simulink library "CPTLibrary"  (R2018a)
settings: Solver=VariableStepAuto  StartTime=0.0  StopTime=10.0  RelTol=1e-3
undefined symbols (not defined in the file or in its folder): DiscIntNeverNeededParam
libraries: $bdroot x28
settings Model: Creator=daniemot  LastModifiedBy=daniemot

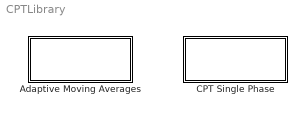
== system CPTLibrary ==
  Adaptive Moving Averages : Subsystem
  CPT Single Phase : Subsystem

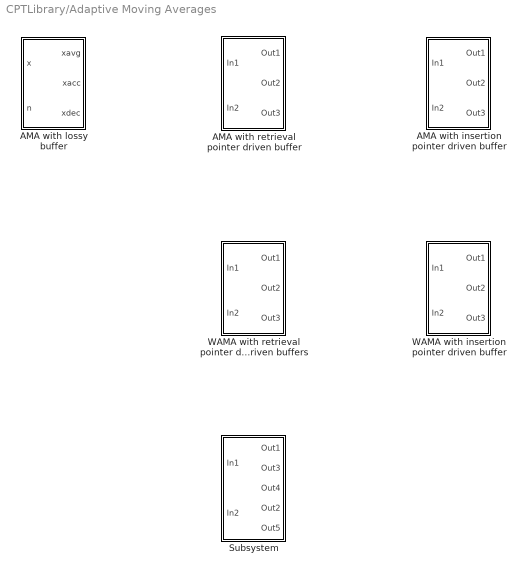
== system CPTLibrary/Adaptive Moving Averages ==
  AMA with insertion pointer driven buffer : Subsystem  TreatAsAtomicUnit=on  SystemSampleTime=Ts  mask(AMA with insertion pointer driven){NbSize=100, Ts=0.001}
      mask prompts: NbSize "Max number of samples for averaging"; Ts "Sampling time [s]"
      mask help:
      | Adaptive moving average with insertion pointer driven circular buffer
      |
      | Interface
      | Input	x (scalar): signal for averaging
      | 	n (scalar): number of previous samples of the input to be averaged with the current input
      | Output	xavg (scalar): average of the current input and the last n-samples of the input.
      | 	xacc (scalar): internal value sent for accumulation
      | 	xdec (scalar): internal value sent for decumulation
      | Parameters	nmax (scalar): maximum length of the length of the circular buffer
      | 	Ts (scalar): sampling time in [s]
      | Internal circular buffer:
      | 	Insertion pointer: i, always marches forward, x(now) replaces the slot pointed by i
      | 	Retrieval pointer: r, lags i by n samples, zeros the slot once retrieved, allowed to jump backwards, collects all values for decumulation and zeros slots when jumping forward.
      |
      | Prog/rev. semi-history:
      | 	Mota, 2020-11-24: first release
  AMA with lossy buffer : Subsystem  TreatAsAtomicUnit=on  SystemSampleTime=Ts  mask(AMA with a skipping circular buffer.){NbSize=100, Ts=0.001}
      mask prompts: NbSize "Max number of samples for averaging"; Ts "Sampling time [s]"
      mask help:
      | Adaptive moving average built with Matlab's discrete variable time delay
      |
      | Interface
      | Input	x (scalar): signal for averaging
      | 	n (scalar): number of previous samples of the input to be averaged with the current input
      | Output	xavg (scalar): average of the current input and the last n-samples of the input.
      | 	xacc (scalar): internal value sent for accumulation
      | 	xdec (scalar): internal value sent for decumulation
      | Parameters	nmax (scalar): maximum length of the length of the circular buffer
      | 	Ts (scalar): sampling time in [s]
      | Internal circular buffer:
      | 	Matlab's variable discrete time delay
      | 	Skips/double decumulations when n changes
      |
      | Prog/rev. semi-history:
      | 	Mota, 2020-11-24: first release
  AMA with retrieval pointer driven buffer : Subsystem  TreatAsAtomicUnit=on  SystemSampleTime=Ts  mask(AMA with retrieval pointer driven buffer){NbSize=100, Ts=0.001}
      mask prompts: NbSize "Max number of samples for averaging"; Ts "Sampling time [s]"
      mask help:
      | Adaptive moving average with retrieval poitner driven circular buffer
      |
      | Interface
      | Input	x (scalar): signal for averaging
      | 	n (scalar): number of previous samples of the input to be averaged with the current input
      | Output	xavg (scalar): average of the current input and the last n-samples of the input.
      | 	xacc (scalar): internal value sent for accumulation
      | 	xdec (scalar): internal value sent for decumulation
      | Parameters	nmax (scalar): maximum length of the length of the circular buffer
      | 	Ts (scalar): sampling time in [s]
      | Internal circular buffer:
      | 	Retrieval pointer: r, always marches forward, zero the slot after retrieval.
      | 	Insertion pointer: i, marches n slots ahead of r, allowed to jump, sums x(now) to the whichever value present at the insertion slot
      |
      | Prog/rev. semi-history:
      | 	Mota, 2020-11-24: first release
  Subsystem : Subsystem  TreatAsAtomicUnit=on  SystemSampleTime=Ts  mask(HAMA with retrieval pointer driven buffer){NbSize=100, Ts=0.001}
      mask prompts: NbSize "Max number of samples for averaging"; Ts "Sampling time [s]"
      mask help:
      | Hybrid adaptive moving average with three retrieval pointer driven circular buffers.
      |
      | Interface
      | Input	x (scalar): signal for averaging
      | 	n (scalar): number of previous samples of the input to be averaged with the current input
      | Output	xavg (scalar): average of the current input and the last hybrid number of 'n'-samples of the input.
      | 	xavground (scalar): average of the current input and the last round(n)-samples of the input.
      | 	xavgceil (scalar): average of the current input and the last ceil(n)-samples of the input.
      | 	xavgfloor (scalar): average of the current input and the last floor(n)-samples of the input.
      | 	xavgweighed (scalar): average of the current input and the last weighted(n)-samples of the input.
      | Parameters	nmax (scalar): maximum length of the length of the circular buffer
      | 	Ts (scalar): sampling time in [s]
      |
      | Prog/rev. semi-history:
      | 	Mota, 2020-12-08: first release
  WAMA with insertion pointer driven buffer : Subsystem  TreatAsAtomicUnit=on  SystemSampleTime=Ts  mask(WAMA with insertion pointer driven buffer){NbSize=0, Ts=0}
      mask prompts: NbSize "Max number of samples for averaging"; Ts "Sampling time [s]"
      mask help:
      | Adaptive moving average with two insertion pointer driven circular buffers.
      |
      | Interface
      | Input	x (scalar): signal for averaging
      | 	n (scalar): number of previous samples of the input to be averaged with the current input
      | Output	xavg (scalar): weigthed average of the current input and the last 'n'-samples of the input.
      | 	xavgceil (scalar): average of the current input and the last ceil(n)-samples of the input.
      | 	xavgfloor (scalar): average of the current input and the last floor(n)-samples of the input.
      | Parameters	nmax (scalar): maximum length of the length of the circular buffer
      | 	Ts (scalar): sampling time in [s]
      |
      | Prog/rev. semi-history:
      | 	Mota, 2020-11-24: first release
  WAMA with retrieval pointer driven buffers : Subsystem  TreatAsAtomicUnit=on  SystemSampleTime=Ts  mask(WAMA with retrieval pointer driven buffer){NbSize=100, Ts=0.001}
      mask prompts: NbSize "Max number of samples for averaging"; Ts "Sampling time [s]"
      mask help:
      | Adaptive moving average with two retrieval pointer driven circular buffers.
      |
      | Interface
      | Input	x (scalar): signal for averaging
      | 	n (scalar): number of previous samples of the input to be averaged with the current input
      | Output	xavg (scalar): weigthed average of the current input and the last 'n'-samples of the input.
      | 	xavgceil (scalar): average of the current input and the last ceil(n)-samples of the input.
      | 	xavgfloor (scalar): average of the current input and the last floor(n)-samples of the input.
      | Parameters	nmax (scalar): maximum length of the length of the circular buffer
      | 	Ts (scalar): sampling time in [s]
      |
      | Prog/rev. semi-history:
      | 	Mota, 2020-11-24: first release

== system CPTLibrary/CPT Single Phase ==
  Single phase CPT Lossy AMA : Subsystem  TreatAsAtomicUnit=on  SystemSampleTime=Ts  mask(Single phase CPT transducer with Skipping AMAs){NbSize=100, Ts=0.001}
      mask prompts: NbSize "Maximum number of samples per period"; Ts "Sampling time [s]"
      mask help:
      | Input	Voltage: v, scalar
      | 	Current: i, scalar
      | 	Frequecy: f, scalar in [Hz]
      | Output	Active power: p
      | 	Active current: ia
      | 	Reactive power: q
      | 	Reactive energy: w
      | 	Reactive current: ir
      | 	Void current: iv
      | 	Integral of the voltage: vint
      | 	Bias of the int. of the volt.: vintbias
      | 	Voltage times current: vi
      | 	Unbiased int. voltage times current: vinthati
      | Parameters	nmax (scalar): maximum length of the length of the circular buffers
      | 	Ts (scalar): sampling time in [s]
      |
      | Prog/rev. semi-history:
      | 	Mota, 2020-11-24: first release
      | 	Mota, 2020-12-08: added voltages and currents to interface
  Single phase CPT Retrieval AMA : Subsystem  TreatAsAtomicUnit=on  SystemSampleTime=Ts  mask(Single Phase CPT Retrieval AMAs){NbSize=100, Ts=0.001}
      mask prompts: NbSize "Maximum number of samples per period"; Ts "Sampling time [s]"
      mask help:
      | Input	Voltage: v, scalar
      | 	Current: i, scalar
      | 	Frequecy: f, scalar in [Hz]
      | Output	Active power: p
      | 	Active current: ia
      | 	Reactive power: q
      | 	Reactive energy: w
      | 	Reactive current: ir
      | 	Void current: iv
      | 	Integral of the voltage: vint
      | 	Bias of the int. of the volt.: vintbias
      | 	Voltage times current: vi
      | 	Unbiased int. voltage times current: vinthati
      | Parameters	nmax (scalar): maximum length of the length of the circular buffers
      | 	Ts (scalar): sampling time in [s]
      |
      | Prog/rev. semi-history:
      | 	Mota, 2020-11-24: first release
      | 	Mota, 2020-12-08: added voltages and currents to interface
  Single phase CPT Retrieval HAMA : Subsystem  TreatAsAtomicUnit=on  SystemSampleTime=Ts  mask{NbSize=100, Ts=0.001}
      mask prompts: NbSize "Maximum number of samples per period"; Ts "Sampling time [s]"
      mask help:
      | Input	Voltage: v, scalar
      | 	Current: i, scalar
      | 	Frequecy: f, scalar in [Hz]
      | Output	Active power: p
      | 	Active current: ia
      | 	Reactive power: q
      | 	Reactive energy: w
      | 	Reactive current: ir
      | 	Void current: iv
      | 	Integral of the voltage: vint
      | 	Bias of the int. of the volt.: vintbias
      | 	Voltage times current: vi
      | 	Unbiased int. voltage times current: vinthati
      | Parameters	nmax (scalar): maximum length of the length of the circular buffers
      | 	Ts (scalar): sampling time in [s]
      |
      | Prog/rev. semi-history:
      | 	Mota, 2020-12-08: first release
  Single phase CPT Retrieval WAMA : Subsystem  TreatAsAtomicUnit=on  SystemSampleTime=Ts  mask(Single phase CPT with Retrieval WAMAs){NbSize=100, Ts=0.001}
      mask prompts: NbSize "Maximum number of samples per period"; Ts "Sampling time [s]"
      mask help:
      | Input	Voltage: v, scalar
      | 	Current: i, scalar
      | 	Frequecy: f, scalar in [Hz]
      | Output	Active power: p
      | 	Active current: ia
      | 	Reactive power: q
      | 	Reactive energy: w
      | 	Reactive current: ir
      | 	Void current: iv
      | 	Integral of the voltage: vint
      | 	Bias of the int. of the volt.: vintbias
      | 	Voltage times current: vi
      | 	Unbiased int. voltage times current: vinthati
      | Parameters	nmax (scalar): maximum length of the length of the circular buffers
      | 	Ts (scalar): sampling time in [s]
      |
      | Prog/rev. semi-history:
      | 	Mota, 2020-11-24: first release
      | 	Mota, 2020-12-08: added voltages and currents to interface

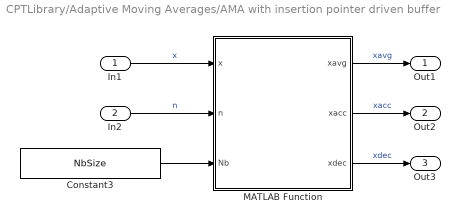
== system CPTLibrary/Adaptive Moving Averages/AMA with insertion pointer driven buffer ==
  In1 : Inport
  In2 : Inport  Port=2
  Constant3 : Constant  Value=NbSize
  MATLAB Function : MATLAB Function  TreatAsAtomicUnit=on
  Out1 : Outport
  Out2 : Outport  Port=2
  Out3 : Outport  Port=3
  wires:
  In2/1 -> MATLAB Function/2(n)  "n"
  MATLAB Function/1(xavg) -> Out1/1  "xavg"
  Constant3/1 -> MATLAB Function/3(Nb)
  MATLAB Function/2(xacc) -> Out2/1  "xacc"
  MATLAB Function/3(xdec) -> Out3/1  "xdec"
  In1/1 -> MATLAB Function/1(x)  "x"

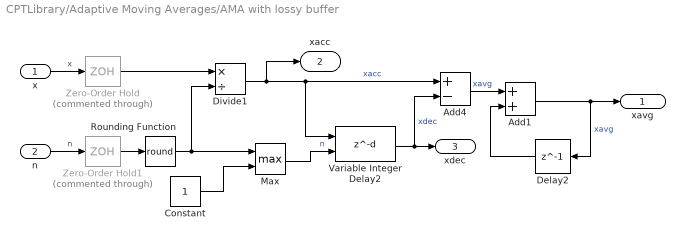
== system CPTLibrary/Adaptive Moving Averages/AMA with lossy buffer ==
  x : Inport
  n : Inport  Port=2
  Add1 : Sum
  Add4 : Sum  Inputs=+-
  Constant : Constant
  Delay2 : Delay  DelayLength=1  InitialCondition=0  UseCircularBuffer=on  SampleTime=Ts
  Divide1 : Product  Inputs=*/
  Max : MinMax  Function=max  Inputs=2
  Rounding Function : Rounding  Operator=round
  Variable Integer Delay2 : Delay  DelayLengthSource=Input port  DelayLengthUpperLimit=NbSize  UseCircularBuffer=on  SampleTime=Ts
      settings: InputPortMap=u0,p1
  Zero-Order Hold : ZeroOrderHold  Commented=through  SampleTime=Ts
  Zero-Order Hold1 : ZeroOrderHold  Commented=through  SampleTime=Ts
  xavg : Outport
  xacc : Outport  Port=2
  xdec : Outport  Port=3
  wires:
  n/1 -> Zero-Order Hold1/1  "n"
  x/1 -> Zero-Order Hold/1  "x"
  Divide1/1 -> Add4/1, Variable Integer Delay2/1, xacc/1  "xacc"
  Variable Integer Delay2/1 -> Add4/2, xdec/1  "xdec"
  Constant/1 -> Max/2
  Max/1 -> Variable Integer Delay2/2  "n"
  Add4/1 -> Add1/1  "xavg"
  Add1/1 -> Delay2/1, xavg/1  "xavg"
  Delay2/1 -> Add1/2
  Zero-Order Hold/1 -> Divide1/1
  Zero-Order Hold1/1 -> Rounding Function/1
  Rounding Function/1 -> Divide1/2, Max/1

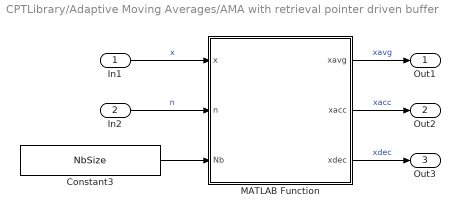
== system CPTLibrary/Adaptive Moving Averages/AMA with retrieval pointer driven buffer ==
  In1 : Inport
  In2 : Inport  Port=2
  Constant3 : Constant  Value=NbSize
  MATLAB Function : MATLAB Function  TreatAsAtomicUnit=on
  Out1 : Outport
  Out2 : Outport  Port=2
  Out3 : Outport  Port=3
  wires:
  MATLAB Function/3(xdec) -> Out3/1  "xdec"
  MATLAB Function/1(xavg) -> Out1/1  "xavg"
  Constant3/1 -> MATLAB Function/3(Nb)
  In1/1 -> MATLAB Function/1(x)  "x"
  In2/1 -> MATLAB Function/2(n)  "n"
  MATLAB Function/2(xacc) -> Out2/1  "xacc"

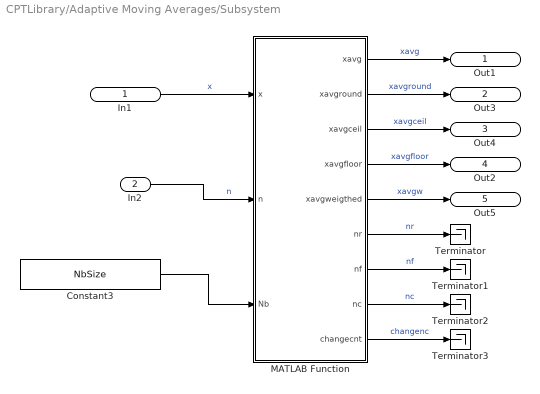
== system CPTLibrary/Adaptive Moving Averages/Subsystem ==
  In1 : Inport
  In2 : Inport  Port=2
  Constant3 : Constant  Value=NbSize
  MATLAB Function : MATLAB Function  TreatAsAtomicUnit=on
  Terminator{,1..3} (4 alike) : Terminator
  Out1 : Outport
  Out3 : Outport  Port=2
  Out4 : Outport  Port=3
  Out2 : Outport  Port=4
  Out5 : Outport  Port=5
  wires:
  MATLAB Function/1(xavg) -> Out1/1  "xavg"
  MATLAB Function/2(xavground) -> Out3/1  "xavground"
  MATLAB Function/3(xavgceil) -> Out4/1  "xavgceil"
  MATLAB Function/4(xavgfloor) -> Out2/1  "xavgfloor"
  MATLAB Function/6(nr) -> Terminator/1  "nr"
  MATLAB Function/7(nf) -> Terminator1/1  "nf"
  MATLAB Function/8(nc) -> Terminator2/1  "nc"
  MATLAB Function/9(changecnt) -> Terminator3/1  "changenc"
  In1/1 -> MATLAB Function/1(x)  "x"
  Constant3/1 -> MATLAB Function/3(Nb)
  In2/1 -> MATLAB Function/2(n)  "n"
  MATLAB Function/5(xavgweigthed) -> Out5/1  "xavgw"

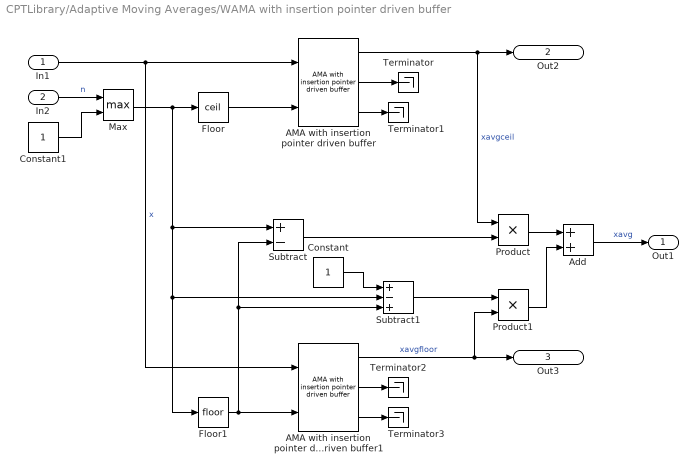
== system CPTLibrary/Adaptive Moving Averages/WAMA with insertion pointer driven buffer ==
  In1 : Inport
  In2 : Inport  Port=2
  AMA with insertion pointer driven buffer : $bdroot/Adaptive Moving Averages/AMA with insertion pointer driven buffer  NbSize=NbSize  Ts=Ts
  AMA with insertion pointer driven buffer1 : $bdroot/Adaptive Moving Averages/AMA with insertion pointer driven buffer  NbSize=NbSize  Ts=Ts
  Add : Sum
  Constant : Constant
  Constant1 : Constant
  Floor : Rounding  Operator=ceil
  Floor1 : Rounding
  Max : MinMax  Function=max  Inputs=2
  Product : Product
  Product1 : Product
  Subtract : Sum  Inputs=+-
  Subtract1 : Sum  Inputs=+-+
  Terminator{,1..3} (4 alike) : Terminator
  Out1 : Outport
  Out2 : Outport  Port=2
  Out3 : Outport  Port=3
  wires:
  AMA with insertion pointer driven buffer/1 -> Out2/1, Product/1  "xavgceil"
  AMA with insertion pointer driven buffer/2 -> Terminator/1
  Floor1/1 -> AMA with insertion pointer driven buffer1/2, Subtract1/3, Subtract/2
  Product1/1 -> Add/2
  Subtract/1 -> Product/2
  Product/1 -> Add/1
  Add/1 -> Out1/1  "xavg"
  Subtract1/1 -> Product1/1
  AMA with insertion pointer driven buffer1/2 -> Terminator2/1
  AMA with insertion pointer driven buffer1/3 -> Terminator3/1
  Floor/1 -> AMA with insertion pointer driven buffer/2
  AMA with insertion pointer driven buffer1/1 -> Product1/2, Out3/1  "xavgfloor"
  AMA with insertion pointer driven buffer/3 -> Terminator1/1
  Constant1/1 -> Max/2
  Max/1 -> Floor1/1, Subtract1/2, Subtract/1, Floor/1
  In2/1 -> Max/1  "n"
  Constant/1 -> Subtract1/1
  In1/1 -> AMA with insertion pointer driven buffer1/1, AMA with insertion pointer driven buffer/1  "x"

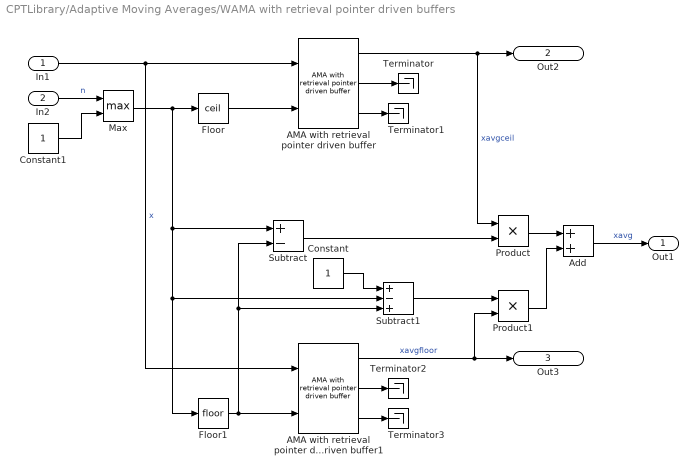
== system CPTLibrary/Adaptive Moving Averages/WAMA with retrieval pointer driven buffers ==
  In1 : Inport
  In2 : Inport  Port=2
  AMA with retrieval pointer driven buffer : $bdroot/Adaptive Moving Averages/AMA with retrieval pointer driven buffer  NbSize=NbSize  Ts=Ts
  AMA with retrieval pointer driven buffer1 : $bdroot/Adaptive Moving Averages/AMA with retrieval pointer driven buffer  NbSize=NbSize  Ts=Ts
  Add : Sum
  Constant : Constant
  Constant1 : Constant
  Floor : Rounding  Operator=ceil
  Floor1 : Rounding
  Max : MinMax  Function=max  Inputs=2
  Product : Product
  Product1 : Product
  Subtract : Sum  Inputs=+-
  Subtract1 : Sum  Inputs=+-+
  Terminator{,1..3} (4 alike) : Terminator
  Out1 : Outport
  Out2 : Outport  Port=2
  Out3 : Outport  Port=3
  wires:
  AMA with retrieval pointer driven buffer/3 -> Terminator1/1
  In1/1 -> AMA with retrieval pointer driven buffer1/1, AMA with retrieval pointer driven buffer/1  "x"
  Floor1/1 -> AMA with retrieval pointer driven buffer1/2, Subtract1/3, Subtract/2
  AMA with retrieval pointer driven buffer/2 -> Terminator/1
  Product1/1 -> Add/2
  Subtract1/1 -> Product1/1
  Add/1 -> Out1/1  "xavg"
  Product/1 -> Add/1
  Subtract/1 -> Product/2
  AMA with retrieval pointer driven buffer/1 -> Out2/1, Product/1  "xavgceil"
  Floor/1 -> AMA with retrieval pointer driven buffer/2
  In2/1 -> Max/1  "n"
  AMA with retrieval pointer driven buffer1/2 -> Terminator2/1
  Constant/1 -> Subtract1/1
  AMA with retrieval pointer driven buffer1/1 -> Product1/2, Out3/1  "xavgfloor"
  AMA with retrieval pointer driven buffer1/3 -> Terminator3/1
  Constant1/1 -> Max/2
  Max/1 -> Floor1/1, Subtract1/2, Subtract/1, Floor/1

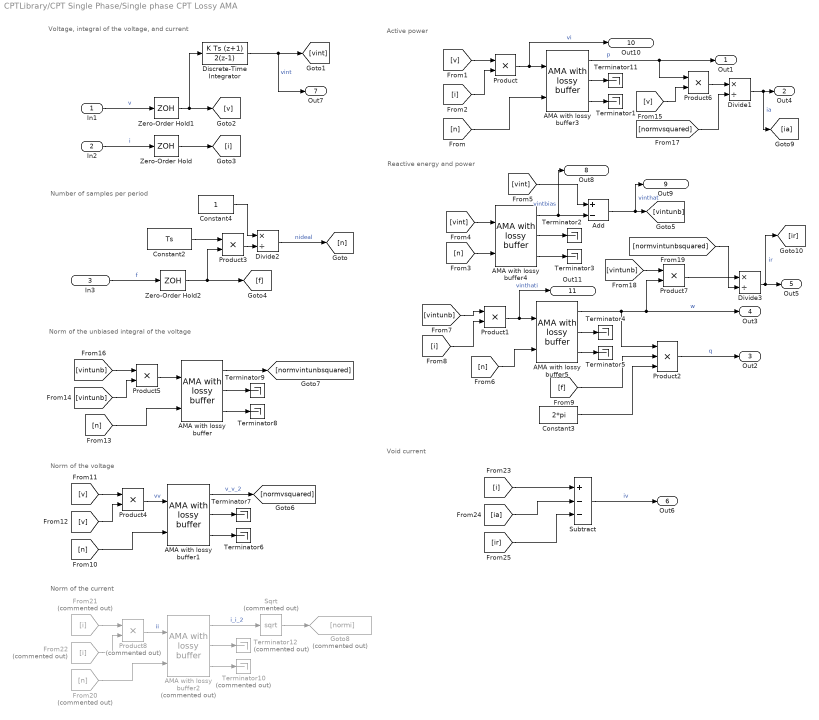
== system CPTLibrary/CPT Single Phase/Single phase CPT Lossy AMA ==
  note: Voltage, integral of the voltage, and current
  note: Number of samples per period
  note: Norm of the unbiased integral of the voltage
  note: Norm of the voltage
  note: Active power
  note: Reactive energy and power
  note: Norm of the current
  note: Void current
  In1 : Inport
  In2 : Inport  Port=2
  In3 : Inport  Port=3
  AMA with lossy buffer{,1,3..5} (5 alike) : $bdroot/Adaptive Moving Averages/AMA with lossy buffer  NbSize=NbSize  Ts=Ts
  AMA with lossy buffer2 : $bdroot/Adaptive Moving Averages/AMA with lossy buffer  Commented=on  NbSize=NbSize  Ts=Ts
  Add : Sum  Inputs=+-
  Constant2 : Constant  Value=Ts
  Constant3 : Constant  Value=2*pi
  Constant4 : Constant
  Discrete-Time Integrator : DiscreteIntegrator  IntegratorMethod=Integration: Trapezoidal  SampleTime=Ts  ICPrevOutput=DiscIntNeverNeededParam  ICPrevScaledInput=DiscIntNeverNeededParam
  Divide1 : Product  Inputs=*/
  Divide2 : Product  Inputs=*/
  Divide3 : Product  Inputs=*/
  From20 : From  Commented=on  GotoTag=n
  From21 : From  Commented=on  GotoTag=i
  From22 : From  Commented=on  GotoTag=i
  Goto8 : Goto  Commented=on  GotoTag=normi
  Product{,1,3..7} (7 alike) : Product
  Product2 : Product  Inputs=3
  Product8 : Product  Commented=on
  Sqrt : Sqrt  Commented=on  SaturateOnIntegerOverflow=on
  Subtract : Sum  Inputs=+--
  Terminator{1..9,11} (10 alike) : Terminator
  Terminator10 : Terminator  Commented=on
  Terminator12 : Terminator  Commented=on
  Zero-Order Hold : ZeroOrderHold  SampleTime=Ts
  Zero-Order Hold1 : ZeroOrderHold  SampleTime=Ts
  Zero-Order Hold2 : ZeroOrderHold  SampleTime=Ts
  Out1 : Outport
  Out4 : Outport  Port=2
  Out2 : Outport  Port=3
  Out3 : Outport  Port=4
  Out5 : Outport  Port=5
  Out6 : Outport  Port=6
  Out7 : Outport  Port=7
  Out8 : Outport  Port=8
  Out9 : Outport  Port=9
  Out10 : Outport  Port=10
  Out11 : Outport  Port=11
  wires:
  [n] -> AMA with lossy buffer3/2
  AMA with lossy buffer3/2 -> Terminator11/1
  AMA with lossy buffer3/3 -> Terminator1/1
  Product1/1 -> Out11/1, AMA with lossy buffer5/1  "vinthati"
  AMA with lossy buffer4/1 -> Out8/1, Add/2  "vintbias"
  AMA with lossy buffer4/2 -> Terminator2/1
  [n] -> AMA with lossy buffer4/2
  AMA with lossy buffer5/3 -> Terminator5/1
  AMA with lossy buffer4/3 -> Terminator3/1
  [n] -> AMA with lossy buffer5/2
  AMA with lossy buffer5/1 -> Product7/2, Out3/1, Product2/1  "w"
  [i] -> Product/2
  In1/1 -> Zero-Order Hold1/1  "v"
  In2/1 -> Zero-Order Hold/1  "i"
  [vint] -> Add/1
  Constant4/1 -> Divide2/1
  Divide2/1 -> [n]  "nideal"
  Product3/1 -> Divide2/2
  [v] -> Product/1
  Constant2/1 -> Product3/1
  AMA with lossy buffer5/2 -> Terminator4/1
  [f] -> Product2/2
  Constant3/1 -> Product2/3
  [i] -> Product1/2
  [vint] -> AMA with lossy buffer4/1
  Zero-Order Hold1/1 -> [v], Discrete-Time Integrator/1
  AMA with lossy buffer3/1 -> Product6/1, Out1/1  "p"
  [vintunb] -> Product1/1
  In3/1 -> Zero-Order Hold2/1  "f"
  Product/1 -> Out10/1, AMA with lossy buffer3/1  "vi"
  Zero-Order Hold2/1 -> Product3/2, [f]
  Zero-Order Hold/1 -> [i]
  Product2/1 -> Out2/1  "q"
  Discrete-Time Integrator/1 -> Out7/1, [vint]  "vint"
  Add/1 -> Out9/1, [vintunb]  "vinthat"
  AMA with lossy buffer1/3 -> Terminator6/1
  AMA with lossy buffer1/2 -> Terminator7/1
  AMA with lossy buffer1/1 -> [normvsquared]  "v_v_2"
  [v] -> Product4/1
  [n] -> AMA with lossy buffer1/2
  Product4/1 -> AMA with lossy buffer1/1  "vv"
  [v] -> Product4/2
  [n] -> AMA with lossy buffer/2
  AMA with lossy buffer/2 -> Terminator9/1
  AMA with lossy buffer/1 -> [normvintunbsquared]
  [vintunb] -> Product5/1
  Product5/1 -> AMA with lossy buffer/1
  AMA with lossy buffer/3 -> Terminator8/1
  [vintunb] -> Product5/2
  [v] -> Product6/2
  Product6/1 -> Divide1/1
  [normvsquared] -> Divide1/2
  Divide1/1 -> [ia], Out4/1  "ia"
  [vintunb] -> Product7/1
  Product7/1 -> Divide3/1
  [normvintunbsquared] -> Divide3/2
  Divide3/1 -> [ir], Out5/1  "ir"
  From20/1 -> AMA with lossy buffer2/2
  AMA with lossy buffer2/2 -> Terminator12/1
  AMA with lossy buffer2/1 -> Sqrt/1  "i_i_2"
  From21/1 -> Product8/1
  Product8/1 -> AMA with lossy buffer2/1  "ii"
  AMA with lossy buffer2/3 -> Terminator10/1
  From22/1 -> Product8/2
  Sqrt/1 -> Goto8/1
  [i] -> Subtract/1
  [ia] -> Subtract/2
  [ir] -> Subtract/3
  Subtract/1 -> Out6/1  "iv"

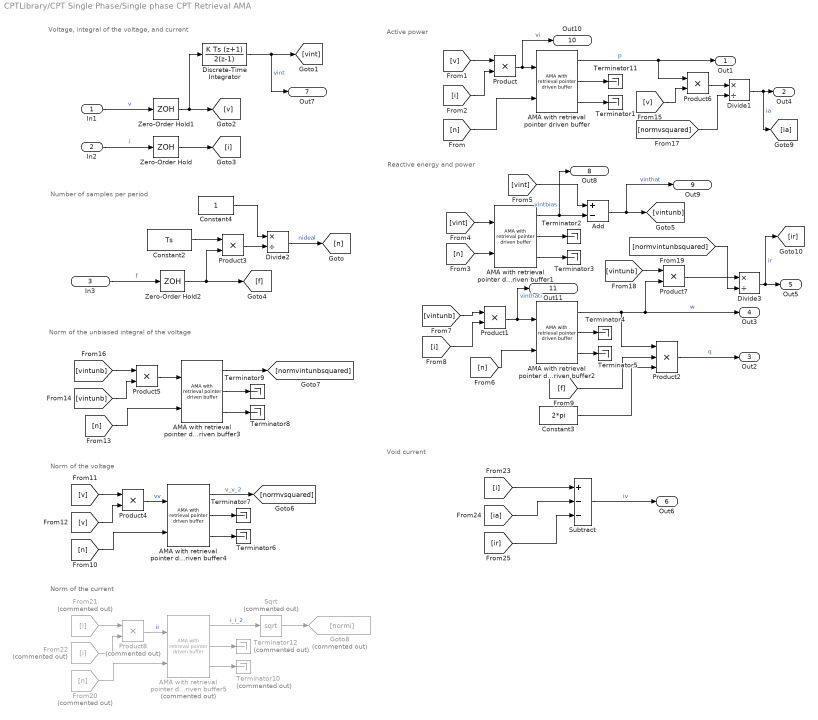
== system CPTLibrary/CPT Single Phase/Single phase CPT Retrieval AMA ==
  note: Norm of the voltage
  note: Void current
  note: Active power
  note: Norm of the current
  note: Number of samples per period
  note: Norm of the unbiased integral of the voltage
  note: Reactive energy and power
  note: Voltage, integral of the voltage, and current
  In1 : Inport
  In2 : Inport  Port=2
  In3 : Inport  Port=3
  AMA with retrieval pointer driven buffer{,1..4} (5 alike) : $bdroot/Adaptive Moving Averages/AMA with retrieval pointer driven buffer  NbSize=NbSize  Ts=Ts
  AMA with retrieval pointer driven buffer5 : $bdroot/Adaptive Moving Averages/AMA with retrieval pointer driven buffer  Commented=on  NbSize=NbSize  Ts=Ts
  Add : Sum  Inputs=+-
  Constant2 : Constant  Value=Ts
  Constant3 : Constant  Value=2*pi
  Constant4 : Constant
  Discrete-Time Integrator : DiscreteIntegrator  IntegratorMethod=Integration: Trapezoidal  SampleTime=Ts  ICPrevOutput=DiscIntNeverNeededParam  ICPrevScaledInput=DiscIntNeverNeededParam
  Divide1 : Product  Inputs=*/
  Divide2 : Product  Inputs=*/
  Divide3 : Product  Inputs=*/
  From20 : From  Commented=on  GotoTag=n
  From21 : From  Commented=on  GotoTag=i
  From22 : From  Commented=on  GotoTag=i
  Goto8 : Goto  Commented=on  GotoTag=normi
  Product{,1,3..7} (7 alike) : Product
  Product2 : Product  Inputs=3
  Product8 : Product  Commented=on
  Sqrt : Sqrt  Commented=on  SaturateOnIntegerOverflow=on
  Subtract : Sum  Inputs=+--
  Terminator{1..9,11} (10 alike) : Terminator
  Terminator10 : Terminator  Commented=on
  Terminator12 : Terminator  Commented=on
  Zero-Order Hold : ZeroOrderHold  SampleTime=Ts
  Zero-Order Hold1 : ZeroOrderHold  SampleTime=Ts
  Zero-Order Hold2 : ZeroOrderHold  SampleTime=Ts
  Out1 : Outport
  Out4 : Outport  Port=2
  Out2 : Outport  Port=3
  Out3 : Outport  Port=4
  Out5 : Outport  Port=5
  Out6 : Outport  Port=6
  Out7 : Outport  Port=7
  Out8 : Outport  Port=8
  Out9 : Outport  Port=9
  Out10 : Outport  Port=10
  Out11 : Outport  Port=11
  wires:
  AMA with retrieval pointer driven buffer2/1 -> Product7/2, Out3/1, Product2/1  "w"
  [n] -> AMA with retrieval pointer driven buffer2/2
  [n] -> AMA with retrieval pointer driven buffer1/2
  [i] -> Subtract/1
  AMA with retrieval pointer driven buffer2/3 -> Terminator5/1
  AMA with retrieval pointer driven buffer/2 -> Terminator11/1
  AMA with retrieval pointer driven buffer/1 -> Product6/1, Out1/1  "p"
  Product4/1 -> AMA with retrieval pointer driven buffer4/1  "vv"
  [ia] -> Subtract/2
  [vintunb] -> Product5/1
  Divide3/1 -> [ir], Out5/1  "ir"
  From22/1 -> Product8/2
  Product8/1 -> AMA with retrieval pointer driven buffer5/1  "ii"
  AMA with retrieval pointer driven buffer5/3 -> Terminator10/1
  From21/1 -> Product8/1
  Divide1/1 -> [ia], Out4/1  "ia"
  [normvintunbsquared] -> Divide3/2
  Product7/1 -> Divide3/1
  [n] -> AMA with retrieval pointer driven buffer4/2
  Sqrt/1 -> Goto8/1
  [vintunb] -> Product7/1
  Product1/1 -> Out11/1, AMA with retrieval pointer driven buffer2/1  "vinthati"
  [v] -> Product6/2
  AMA with retrieval pointer driven buffer3/1 -> [normvintunbsquared]
  [normvsquared] -> Divide1/2
  AMA with retrieval pointer driven buffer3/2 -> Terminator9/1
  AMA with retrieval pointer driven buffer2/2 -> Terminator4/1
  AMA with retrieval pointer driven buffer4/1 -> [normvsquared]  "v_v_2"
  [n] -> AMA with retrieval pointer driven buffer3/2
  AMA with retrieval pointer driven buffer4/2 -> Terminator7/1
  Discrete-Time Integrator/1 -> Out7/1, [vint]  "vint"
  Zero-Order Hold/1 -> [i]
  In3/1 -> Zero-Order Hold2/1  "f"
  AMA with retrieval pointer driven buffer/3 -> Terminator1/1
  Zero-Order Hold1/1 -> [v], Discrete-Time Integrator/1
  [vintunb] -> Product1/1
  [i] -> Product1/2
  Constant3/1 -> Product2/3
  [f] -> Product2/2
  [vint] -> Add/1
  [ir] -> Subtract/3
  Constant2/1 -> Product3/1
  Product3/1 -> Divide2/2
  Divide2/1 -> [n]  "nideal"
  [v] -> Product/1
  Zero-Order Hold2/1 -> Product3/2, [f]
  [i] -> Product/2
  In2/1 -> Zero-Order Hold/1  "i"
  In1/1 -> Zero-Order Hold1/1  "v"
  AMA with retrieval pointer driven buffer3/3 -> Terminator8/1
  From20/1 -> AMA with retrieval pointer driven buffer5/2
  Product5/1 -> AMA with retrieval pointer driven buffer3/1
  [n] -> AMA with retrieval pointer driven buffer/2
  [v] -> Product4/1
  [vint] -> AMA with retrieval pointer driven buffer1/1
  AMA with retrieval pointer driven buffer1/2 -> Terminator2/1
  Subtract/1 -> Out6/1  "iv"
  AMA with retrieval pointer driven buffer4/3 -> Terminator6/1
  Product6/1 -> Divide1/1
  AMA with retrieval pointer driven buffer5/1 -> Sqrt/1  "i_i_2"
  Add/1 -> Out9/1, [vintunb]  "vinthat"
  Product/1 -> Out10/1, AMA with retrieval pointer driven buffer/1  "vi"
  AMA with retrieval pointer driven buffer1/3 -> Terminator3/1
  Constant4/1 -> Divide2/1
  [v] -> Product4/2
  [vintunb] -> Product5/2
  Product2/1 -> Out2/1  "q"
  AMA with retrieval pointer driven buffer5/2 -> Terminator12/1
  AMA with retrieval pointer driven buffer1/1 -> Out8/1, Add/2  "vintbias"

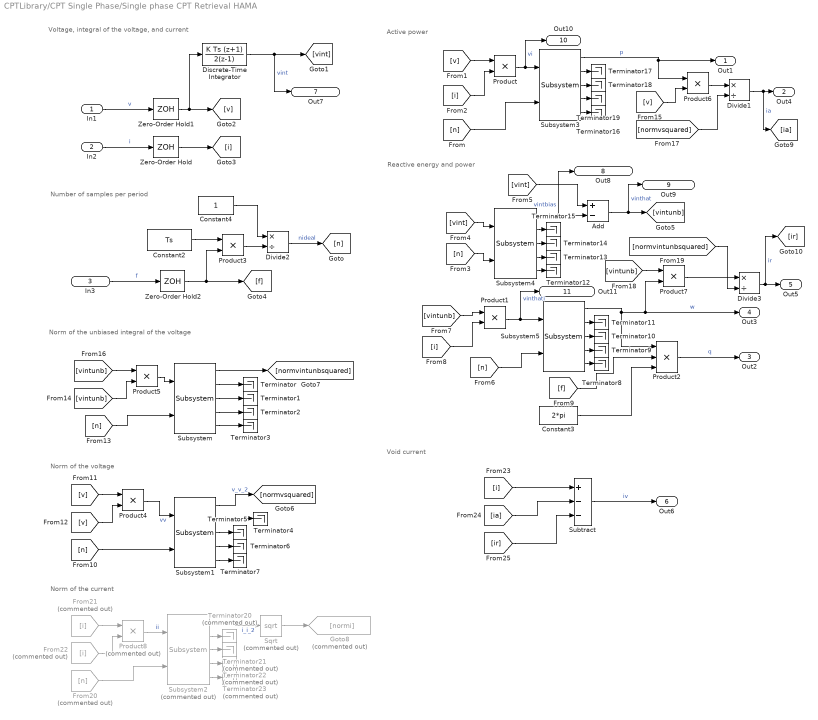
== system CPTLibrary/CPT Single Phase/Single phase CPT Retrieval HAMA ==
  note: Void current
  note: Number of samples per period
  note: Norm of the voltage
  note: Voltage, integral of the voltage, and current
  note: Reactive energy and power
  note: Active power
  note: Norm of the current
  note: Norm of the unbiased integral of the voltage
  In1 : Inport
  In2 : Inport  Port=2
  In3 : Inport  Port=3
  Add : Sum  Inputs=+-
  Constant2 : Constant  Value=Ts
  Constant3 : Constant  Value=2*pi
  Constant4 : Constant
  Discrete-Time Integrator : DiscreteIntegrator  IntegratorMethod=Integration: Trapezoidal  SampleTime=Ts  ICPrevOutput=DiscIntNeverNeededParam  ICPrevScaledInput=DiscIntNeverNeededParam
  Divide1 : Product  Inputs=*/
  Divide2 : Product  Inputs=*/
  Divide3 : Product  Inputs=*/
  From20 : From  Commented=on  GotoTag=n
  From21 : From  Commented=on  GotoTag=i
  From22 : From  Commented=on  GotoTag=i
  Goto8 : Goto  Commented=on  GotoTag=normi
  Product{,1,3..7} (7 alike) : Product
  Product2 : Product  Inputs=3
  Product8 : Product  Commented=on
  Sqrt : Sqrt  Commented=on  SaturateOnIntegerOverflow=on
  Subsystem{,1,3..5} (5 alike) : $bdroot/Adaptive Moving Averages/Subsystem  NbSize=NbSize  Ts=Ts
  Subsystem2 : $bdroot/Adaptive Moving Averages/Subsystem  Commented=on  NbSize=NbSize  Ts=Ts
  Subtract : Sum  Inputs=+--
  Terminator{,1..19} (20 alike) : Terminator
  Terminator{20..23} (4 alike) : Terminator  Commented=on
  Zero-Order Hold : ZeroOrderHold  SampleTime=Ts
  Zero-Order Hold1 : ZeroOrderHold  SampleTime=Ts
  Zero-Order Hold2 : ZeroOrderHold  SampleTime=Ts
  Out1 : Outport
  Out4 : Outport  Port=2
  Out2 : Outport  Port=3
  Out3 : Outport  Port=4
  Out5 : Outport  Port=5
  Out6 : Outport  Port=6
  Out7 : Outport  Port=7
  Out8 : Outport  Port=8
  Out9 : Outport  Port=9
  Out10 : Outport  Port=10
  Out11 : Outport  Port=11
  wires:
  Product6/1 -> Divide1/1
  [i] -> Product/2
  Product3/1 -> Divide2/2
  Product7/1 -> Divide3/1
  [ia] -> Subtract/2
  [f] -> Product2/2
  Divide3/1 -> [ir], Out5/1  "ir"
  Subsystem2/1 -> Sqrt/1  "i_i_2"
  Product8/1 -> Subsystem2/1  "ii"
  [v] -> Product4/1
  Subtract/1 -> Out6/1  "iv"
  In2/1 -> Zero-Order Hold/1  "i"
  In1/1 -> Zero-Order Hold1/1  "v"
  [v] -> Product/1
  [v] -> Product4/2
  [n] -> Subsystem/2
  [vint] -> Add/1
  Add/1 -> Out9/1, [vintunb]  "vinthat"
  From21/1 -> Product8/1
  Subsystem4/1 -> Out8/1, Add/2  "vintbias"
  Zero-Order Hold2/1 -> Product3/2, [f]
  [ir] -> Subtract/3
  Divide2/1 -> [n]  "nideal"
  Product1/1 -> Subsystem5/1, Out11/1  "vinthati"
  Zero-Order Hold/1 -> [i]
  Divide1/1 -> [ia], Out4/1  "ia"
  [vintunb] -> Product7/1
  Product2/1 -> Out2/1  "q"
  Constant3/1 -> Product2/3
  From22/1 -> Product8/2
  [vintunb] -> Product5/1
  [normvintunbsquared] -> Divide3/2
  Discrete-Time Integrator/1 -> Out7/1, [vint]  "vint"
  [vintunb] -> Product5/2
  [i] -> Subtract/1
  Product5/1 -> Subsystem/1
  [vintunb] -> Product1/1
  Subsystem1/1 -> [normvsquared]  "v_v_2"
  Product/1 -> Subsystem3/1, Out10/1  "vi"
  [v] -> Product6/2
  Constant2/1 -> Product3/1
  [i] -> Product1/2
  Product4/1 -> Subsystem1/1  "vv"
  [n] -> Subsystem1/2
  Subsystem5/1 -> Product2/1, Product7/2, Out3/1  "w"
  [normvsquared] -> Divide1/2
  Zero-Order Hold1/1 -> [v], Discrete-Time Integrator/1
  In3/1 -> Zero-Order Hold2/1  "f"
  Constant4/1 -> Divide2/1
  Subsystem/1 -> [normvintunbsquared]
  Sqrt/1 -> Goto8/1
  Subsystem3/1 -> Product6/1, Out1/1  "p"
  From20/1 -> Subsystem2/2
  [n] -> Subsystem3/2
  [vint] -> Subsystem4/1
  [n] -> Subsystem4/2
  [n] -> Subsystem5/2
  Subsystem/2 -> Terminator/1
  Subsystem/3 -> Terminator1/1
  Subsystem/4 -> Terminator2/1
  Subsystem/5 -> Terminator3/1
  Subsystem1/2 -> Terminator4/1
  Subsystem1/3 -> Terminator5/1
  Subsystem1/4 -> Terminator6/1
  Subsystem1/5 -> Terminator7/1
  Subsystem5/5 -> Terminator8/1
  Subsystem5/4 -> Terminator9/1
  Subsystem5/3 -> Terminator10/1
  Subsystem5/2 -> Terminator11/1
  Subsystem4/5 -> Terminator12/1
  Subsystem4/4 -> Terminator13/1
  Subsystem4/3 -> Terminator14/1
  Subsystem4/2 -> Terminator15/1
  Subsystem3/5 -> Terminator16/1
  Subsystem3/2 -> Terminator17/1
  Subsystem3/3 -> Terminator18/1
  Subsystem3/4 -> Terminator19/1
  Subsystem2/2 -> Terminator20/1
  Subsystem2/3 -> Terminator21/1
  Subsystem2/4 -> Terminator22/1
  Subsystem2/5 -> Terminator23/1

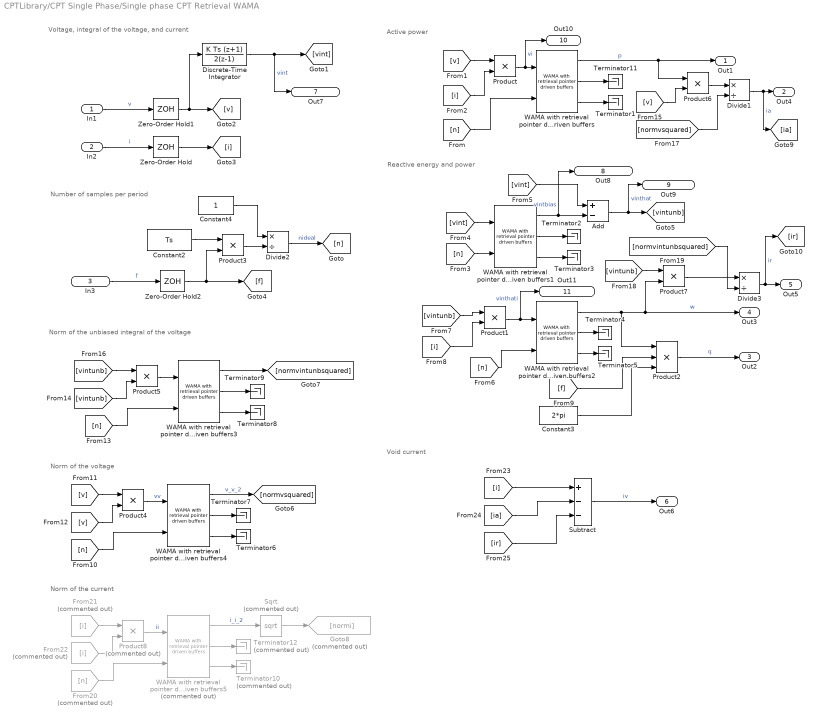
== system CPTLibrary/CPT Single Phase/Single phase CPT Retrieval WAMA ==
  note: Voltage, integral of the voltage, and current
  note: Number of samples per period
  note: Reactive energy and power
  note: Active power
  note: Norm of the voltage
  note: Norm of the unbiased integral of the voltage
  note: Norm of the current
  note: Void current
  In1 : Inport
  In2 : Inport  Port=2
  In3 : Inport  Port=3
  Add : Sum  Inputs=+-
  Constant2 : Constant  Value=Ts
  Constant3 : Constant  Value=2*pi
  Constant4 : Constant
  Discrete-Time Integrator : DiscreteIntegrator  IntegratorMethod=Integration: Trapezoidal  SampleTime=Ts  ICPrevOutput=DiscIntNeverNeededParam  ICPrevScaledInput=DiscIntNeverNeededParam
  Divide1 : Product  Inputs=*/
  Divide2 : Product  Inputs=*/
  Divide3 : Product  Inputs=*/
  From20 : From  Commented=on  GotoTag=n
  From21 : From  Commented=on  GotoTag=i
  From22 : From  Commented=on  GotoTag=i
  Goto8 : Goto  Commented=on  GotoTag=normi
  Product{,1,3..7} (7 alike) : Product
  Product2 : Product  Inputs=3
  Product8 : Product  Commented=on
  Sqrt : Sqrt  Commented=on  SaturateOnIntegerOverflow=on
  Subtract : Sum  Inputs=+--
  Terminator{1..9,11} (10 alike) : Terminator
  Terminator10 : Terminator  Commented=on
  Terminator12 : Terminator  Commented=on
  WAMA with retrieval pointer driven buffers{,1..4} (5 alike) : $bdroot/Adaptive Moving Averages/WAMA with retrieval pointer driven buffers  NbSize=NbSize  Ts=Ts
  WAMA with retrieval pointer driven buffers5 : $bdroot/Adaptive Moving Averages/WAMA with retrieval pointer driven buffers  Commented=on  NbSize=NbSize  Ts=Ts
  Zero-Order Hold : ZeroOrderHold  SampleTime=Ts
  Zero-Order Hold1 : ZeroOrderHold  SampleTime=Ts
  Zero-Order Hold2 : ZeroOrderHold  SampleTime=Ts
  Out1 : Outport
  Out4 : Outport  Port=2
  Out2 : Outport  Port=3
  Out3 : Outport  Port=4
  Out5 : Outport  Port=5
  Out6 : Outport  Port=6
  Out7 : Outport  Port=7
  Out8 : Outport  Port=8
  Out9 : Outport  Port=9
  Out10 : Outport  Port=10
  Out11 : Outport  Port=11
  wires:
  Discrete-Time Integrator/1 -> Out7/1, [vint]  "vint"
  In3/1 -> Zero-Order Hold2/1  "f"
  Zero-Order Hold1/1 -> [v], Discrete-Time Integrator/1
  [i] -> Subtract/1
  WAMA with retrieval pointer driven buffers3/1 -> [normvintunbsquared]
  Product5/1 -> WAMA with retrieval pointer driven buffers3/1
  WAMA with retrieval pointer driven buffers3/2 -> Terminator9/1
  WAMA with retrieval pointer driven buffers3/3 -> Terminator8/1
  Product4/1 -> WAMA with retrieval pointer driven buffers4/1  "vv"
  WAMA with retrieval pointer driven buffers4/3 -> Terminator6/1
  WAMA with retrieval pointer driven buffers4/2 -> Terminator7/1
  WAMA with retrieval pointer driven buffers4/1 -> [normvsquared]  "v_v_2"
  [n] -> WAMA with retrieval pointer driven buffers4/2
  [vint] -> WAMA with retrieval pointer driven buffers1/1
  WAMA with retrieval pointer driven buffers5/3 -> Terminator10/1
  WAMA with retrieval pointer driven buffers1/2 -> Terminator2/1
  WAMA with retrieval pointer driven buffers/2 -> Terminator11/1
  WAMA with retrieval pointer driven buffers/3 -> Terminator1/1
  WAMA with retrieval pointer driven buffers2/2 -> Terminator4/1
  Product1/1 -> Out11/1, WAMA with retrieval pointer driven buffers2/1  "vinthati"
  [v] -> Product6/2
  WAMA with retrieval pointer driven buffers2/1 -> Product7/2, Out3/1, Product2/1  "w"
  Product/1 -> Out10/1, WAMA with retrieval pointer driven buffers/1  "vi"
  [vintunb] -> Product7/1
  [normvsquared] -> Divide1/2
  [normvintunbsquared] -> Divide3/2
  Divide1/1 -> [ia], Out4/1  "ia"
  Zero-Order Hold/1 -> [i]
  [vint] -> Add/1
  Constant3/1 -> Product2/3
  [i] -> Product1/2
  [vintunb] -> Product1/1
  Constant2/1 -> Product3/1
  [vintunb] -> Product5/1
  [ir] -> Subtract/3
  From22/1 -> Product8/2
  [n] -> WAMA with retrieval pointer driven buffers2/2
  WAMA with retrieval pointer driven buffers5/2 -> Terminator12/1
  Zero-Order Hold2/1 -> Product3/2, [f]
  Product7/1 -> Divide3/1
  WAMA with retrieval pointer driven buffers1/3 -> Terminator3/1
  Sqrt/1 -> Goto8/1
  Divide2/1 -> [n]  "nideal"
  WAMA with retrieval pointer driven buffers5/1 -> Sqrt/1  "i_i_2"
  Constant4/1 -> Divide2/1
  Product2/1 -> Out2/1  "q"
  [n] -> WAMA with retrieval pointer driven buffers3/2
  Product3/1 -> Divide2/2
  [n] -> WAMA with retrieval pointer driven buffers/2
  From20/1 -> WAMA with retrieval pointer driven buffers5/2
  [vintunb] -> Product5/2
  [v] -> Product4/2
  Product8/1 -> WAMA with retrieval pointer driven buffers5/1  "ii"
  Product6/1 -> Divide1/1
  WAMA with retrieval pointer driven buffers1/1 -> Out8/1, Add/2  "vintbias"
  Add/1 -> Out9/1, [vintunb]  "vinthat"
  [f] -> Product2/2
  In1/1 -> Zero-Order Hold1/1  "v"
  From21/1 -> Product8/1
  WAMA with retrieval pointer driven buffers/1 -> Product6/1, Out1/1  "p"
  Subtract/1 -> Out6/1  "iv"
  [i] -> Product/2
  In2/1 -> Zero-Order Hold/1  "i"
  [n] -> WAMA with retrieval pointer driven buffers1/2
  Divide3/1 -> [ir], Out5/1  "ir"
  [v] -> Product4/1
  WAMA with retrieval pointer driven buffers2/3 -> Terminator5/1
  [v] -> Product/1
  [ia] -> Subtract/2

== matlab function CPTLibrary/Adaptive Moving Averages/AMA with insertion pointer driven buffer/MATLAB Function ==
  data: x input; xavg output; n input; Nb input; xacc output; xdec output
%%%%%%%%%%%%%%%%%%%%%%%%%%%%%%%%%%%%%%%%%%%%%%%%%%%%%%%%%%%%%%%%%%%%%%%%%%
% Adaptive Moving Average Block
%%%%%%%%%%%%%%%%%%%%%%%%%%%%%%%%%%%%%%%%%%%%%%%%%%%%%%%%%%%%%%%%%%%%%%%%%%
function [xavg, xacc, xdec]  = AMAInsertionPntrDriven( x, n, Nb)

persistent buffer bufferlen rzero izero rone ione Nb_fix xavg_internal nold
 
for_acc_internal = 0;
for_dec_internal = 0;

%%%%%%%%%%%%%%%%%%%%%%%%%%%%%%%%%%
% Values of at the first cycle
%%%%%%%%%%%%%%%%%%%%%%%%%%%%%%%%%%
if isempty(buffer)
    %Nb should be larger than 2
    if Nb < 1
        %lenght of the buffer is Nb+1
        Nb_fix = 1;
        bufferlen = 2;
    else
        Nb_fix = round(Nb); %lenght of the buffer is Nb+1
        bufferlen = Nb_fix + 1;
    end
    
    %create the buffer with zeros 
    buffer = zeros(bufferlen,1);
    
    %check is n smaller or equal to Nb
    if n > Nb_fix
        n = Nb_fix;
    else
        if n < 1
            n = 1; 
        else
            n = round(n);
        end
    end
    
    %initialize pointers
    rzero = 0;
    izero = rzero + n;
    
    rone = rzero + 1;
    ione = izero + 1;
    
    %first insertion 
    %bufferlen = Nb+1 so I can write to the buffer first
    buffer(ione) = x/n;
    
    %calculating value for accumulation
    for_acc_internal = x/n;
    for_dec_internal = 0;
    
    %accumulator
    xavg_internal = for_acc_internal; 
    nold = n;
else
%%%%%%%%%%%%%%%%%%%%%%%%%%%%%%%%%%
% Here the function starts actually
%%%%%%%%%%%%%%%%%%%%%%%%%%%%%%%%%%
    %check if n smaller or equal to Nb
    if n > Nb_fix
        n = Nb_fix;
    else
        if n < 1
            n = 1; 
        else
            n = round(n);
        end
    end
    
    %insertion pointer moves forward, slot is replaced
    %bufferlen = Nb+1 so I can write to the buffer first
    izero = round( mod(izero + 1, bufferlen));
    ione = izero + 1;
    buffer(ione) = x/n;
    for_acc_internal = x/n; 
    
    %retrieval logic
    if n >= nold
        %retrieval pointer can jump backwards (as I had zeroed the buffer
        %after retrievals)
        rzero = round( mod(izero - n, bufferlen));
        rone = rzero + 1;
        for_dec_internal = buffer(rone);
        buffer(rone) = 0;
        nold = n;
    else
        jump = nold - n;
        for aux=0:jump
            rzero = round( mod(rzero + 1, bufferlen));
            rone = rzero + 1;
            for_dec_internal = for_dec_internal + buffer(rone);
            buffer(rone) = 0;
            nold = n;
        end
    end
    
    %accumulation
    xavg_internal = xavg_internal + for_acc_internal - for_dec_internal; 
end

xacc = for_acc_internal;
xdec = for_dec_internal;
xavg = xavg_internal;

== matlab function CPTLibrary/Adaptive Moving Averages/AMA with retrieval pointer driven buffer/MATLAB Function ==
  data: x input; xavg output; n input; Nb input; xacc output; xdec output
%%%%%%%%%%%%%%%%%%%%%%%%%%%%%%%%%%%%%%%%%%%%%%%%%%%%%%%%%%%%%%%%%%%%%%%%%%
% Adaptive Moving Average Block
%%%%%%%%%%%%%%%%%%%%%%%%%%%%%%%%%%%%%%%%%%%%%%%%%%%%%%%%%%%%%%%%%%%%%%%%%%
% Prog/rev history
%   Mota - 2020-11-24: first release
function [xavg, xacc, xdec]  = AMARetrievalPntrDriven( x, n, Nb)

persistent buffer bufferlen r i Nb_fix xavg_internal

for_acc_internal = 0;
for_dec_internal = 0;

%%%%%%%%%%%%%%%%%%%%%%%%%%%%%%%%%%
% Values at the first cycle
%%%%%%%%%%%%%%%%%%%%%%%%%%%%%%%%%%
if isempty(buffer)
    %Nb should be larger than 1
    if Nb < 1
        %lenght of the buffer is Nb+1
        Nb_fix = 1;
        bufferlen = 2;
    else
        Nb_fix = round(Nb); %lenght of the buffer is Nb+1
        bufferlen = Nb_fix + 1;
    end
    
    %create the buffer with zeros 
    buffer = zeros(bufferlen,1);
    
    %check is n smaller or equal to Nb
    if n > Nb_fix
        n = Nb_fix;
    else
        if n < 1
            n = 1; 
        else
            n = round(n);
        end
    end
    
    %initialize pointers
    r = 1;
    i = r + n;
    
    %first sum 
    buffer(i) = buffer(i) + x/n;
    
    %calculating value for accumulation
    for_acc_internal = x/n;
    for_dec_internal = 0;
    
    %accumulator
    %xavg_internal = for_acc_internal - for_dec_internal; %first cycle, for_dec_internal=0
    xavg_internal = for_acc_internal; 
else
%%%%%%%%%%%%%%%%%%%%%%%%%%%%%%%%%%
% Here the function starts actually
%%%%%%%%%%%%%%%%%%%%%%%%%%%%%%%%%%
    %check if n smaller or equal to Nb
    if n > Nb_fix
        n = Nb_fix;
    else
        if n < 1
            n = 1; 
        else
            n = round(n);
        end
    end
    
    %pointer update
    r = r + 1;
    r = round( mod(r - 1, bufferlen) + 1); %mod works with index starting at zero, but matlab works with index on 1 
    i = round( mod(r - 1 + n, bufferlen) + 1);
    
    %insertion (sum)
    for_acc_internal = x/n; 
    buffer(i) = buffer(i) + for_acc_internal;
        
    %retrieval and zeroing 
    for_dec_internal = buffer(r);
    buffer(r) = 0; 
    
    %accumulation
    xavg_internal = xavg_internal + for_acc_internal - for_dec_internal; 
end

xacc = for_acc_internal;
xdec = for_dec_internal;
xavg = xavg_internal;

== matlab function CPTLibrary/Adaptive Moving Averages/Subsystem/MATLAB Function ==
  data: x input; xavg output; xavground output; n input; Nb input; xavgceil output; xavgfloor output; xavgweigthed output; nr output; nf output; nc output; changecnt output
%%%%%%%%%%%%%%%%%%%%%%%%%%%%%%%%%%%%%%%%%%%%%%%%%%%%%%%%%%%%%%%%%%%%%%%%%%
% Adaptive Moving Average Block
%%%%%%%%%%%%%%%%%%%%%%%%%%%%%%%%%%%%%%%%%%%%%%%%%%%%%%%%%%%%%%%%%%%%%%%%%%
% Prog/rev history
%   Mota - 2020-12-08: first release

function [xavg, xavground, xavgceil, xavgfloor, xavgweigthed, nr, nf, nc, changecnt]  = AMARetrievalPntrDriven( x, n, Nb)

persistent bufferlen Nb_fix
persistent bufferround nround rround iround
persistent bufferceil nceil rceil iceil
persistent bufferfloor nfloor rfloor ifloor
persistent xavg_internal_ceil xavg_internal_round xavg_internal_floor
persistent old_nceil k_change_counter

for_acc_internal_ceil = 0;
for_dec_internal_ceil = 0;

for_acc_internal_round = 0;
for_dec_internal_round = 0;

for_acc_internal_floor = 0;
for_dec_internal_floor = 0;

nnow = n; 

%%%%%%%%%%%%%%%%%%%%%%%%%%%%%%%%%%
% Values of at the first cycle
%%%%%%%%%%%%%%%%%%%%%%%%%%%%%%%%%%
if isempty(bufferceil)
    %Nb should be larger than 1
    if Nb < 1
        %lenght of the buffer is Nb+1
        Nb_fix = 1;
        bufferlen = 2;
    else
        Nb_fix = round(Nb);%lenght of the buffer is Nb+1
        bufferlen = round(Nb_fix+1);
    end
    
    %initialize the buffer
    bufferceil = zeros(bufferlen,1);
    bufferround = zeros(bufferlen,1);
    bufferfloor = zeros(bufferlen,1);
    
    %check is n smaller or equal to Nb
    if nnow > Nb_fix
        nnow = Nb_fix;
        nceil = Nb_fix;
        nround = Nb_fix;
        nfloor = Nb_fix;
    else
        if nnow < 1
            nnow = 1;
            nceil = 1;
            nround = 1;
            nfloor = 1;
        else
            nceil = ceil(nnow);
            nround = round(nnow);
            nfloor = floor(nnow);
        end
    end
    
    %detecting change in ceiling
    old_nceil = nceil;
    k_change_counter = 0; 
    
    %initialize pointers
    rceil = 1;
    iceil = rceil + nceil;
    
    rround = 1;
    iround = rround + nround;
        
    rfloor = 1;
    ifloor = rfloor + nfloor;
        
    %first sum 
    bufferceil(iceil) = bufferceil(iceil) + x/nceil;
    bufferround(iround) = bufferround(iround) + x/nround;
    bufferfloor(ifloor) = bufferfloor(ifloor) + x/nfloor;
    
    %calculating value for accumulation
    for_acc_internal_ceil  = x/nceil;
    for_dec_internal_ceil = 0;
    
    for_acc_internal_round  = x/nround;
    for_dec_internal_round = 0;        
    
    for_acc_internal_floor  = x/nfloor;
    for_dec_internal_floor = 0;
        
    %accumulator
    xavg_internal_ceil = for_acc_internal_ceil; 
    xavg_internal_round = for_acc_internal_round; 
    xavg_internal_floor = for_acc_internal_floor; 
else
%%%%%%%%%%%%%%%%%%%%%%%%%%%%%%%%%%
% Here the function starts actually
%%%%%%%%%%%%%%%%%%%%%%%%%%%%%%%%%%
    %check is n smaller or equal to Nb
    if nnow > Nb_fix
        nnow = Nb_fix;
        nceil = Nb_fix;
        nround = Nb_fix;
        nfloor = Nb_fix;
    else
        if nnow < 1
            nnow = 1;
            nceil = 1;
            nround = 1;
            nfloor = 1;
        else
            nceil = ceil(nnow);
            nround = round(nnow);
            nfloor = floor(nnow);
        end
    end
    
    %pointer update
    %mod works from zero, matlab arrays start at index 1
    rceil = rceil + 1;
    rceil = round( mod(rceil - 1, bufferlen)+1); 
    iceil = round( mod(rceil - 1 + nceil, bufferlen) + 1);

    rround = rround + 1;
    rround = round( mod(rround - 1, bufferlen)+1); 
    iround = round( mod(rround - 1 + nround, bufferlen) + 1);
    
    rfloor = rfloor + 1;
    rfloor = round( mod(rfloor - 1, bufferlen)+1); 
    ifloor = round( mod(rfloor - 1 + nfloor, bufferlen) + 1);

    %insertion (sum)
    for_acc_internal_ceil = x/nceil; 
    bufferceil(iceil) = bufferceil(iceil) + for_acc_internal_ceil;

    for_acc_internal_round = x/nround; 
    bufferround(iround) = bufferround(iround) + for_acc_internal_round;
    
    for_acc_internal_floor = x/nfloor; 
    bufferfloor(ifloor) = bufferfloor(ifloor) + for_acc_internal_floor;

    
    %retrieval and zeroing 
    for_dec_internal_ceil = bufferceil(rceil);
    bufferceil(rceil) = 0; 

    for_dec_internal_round = bufferround(rround);
    bufferround(rround) = 0; 
        
    for_dec_internal_floor = bufferfloor(rfloor);
    bufferfloor(rfloor) = 0; 
    
    
    %accumulation
    xavg_internal_ceil = xavg_internal_ceil + for_acc_internal_ceil - for_dec_internal_ceil; 
    xavg_internal_round = xavg_internal_round + for_acc_internal_round - for_dec_internal_round; 
    xavg_internal_floor = xavg_internal_floor + for_acc_internal_floor - for_dec_internal_floor; 
end

xavgceil = xavg_internal_ceil;
xavground = xavg_internal_round;
xavgfloor = xavg_internal_floor;
xavgweigthed = (nnow - nfloor) * xavg_internal_ceil + (1 - nnow + nfloor) * xavg_internal_floor;
%alpha = (nnow - nfloor);
%oneminusalpha = (1 - nnow + nfloor);

nr = nround;
nf = nfloor;
nc = nceil;
changenc = 0;

%Check for changes in nceil and start a timer
if old_nceil ~= nceil
    changenc = 1;
    k_change_counter = 1; 
else
    if k_change_counter > 0
        k_change_counter = k_change_counter  + 1;
        if k_change_counter > nceil
            changenc = 0; 
            k_change_counter = 0;
        else
            changenc = 1;
        end
    end
end

if changenc == 1
    xavg = xavg_internal_round;
else
    xavg = (nnow - nfloor) * xavg_internal_ceil + (1 - nnow + nfloor) * xavg_internal_floor;
end
old_nceil = nceil;
changecnt = k_change_counter;
